simulink subsystem "sdf_node"  (R2022b)
settings: Solver=VariableStepAuto  StartTime=0.0  StopTime=10.0  RelTol=1e-3
model mask{Parameter1=0, Parameter2=0, Parameter3=0, Parameter4=0}
  mask prompts: Parameter1 "alpha"; Parameter2 "beta"; Parameter3 "k"; Parameter4 "Accumulator"
settings Model: Creator=1111293  LastModifiedBy=qaztr
settings SolverCC: AlgebraicLoopSolver=TrustRegion
settings DebuggingCC: UnconnectedInputMsg=warning  UnconnectedOutputMsg=warning  UnconnectedLineMsg=warning  SFMachineParentedDataDiag=warning
settings ModelReferenceCC: EnableRefExpFcnMdlSchedulingChecks=on
settings RTWCC: DLArmComputeVersion=19.05

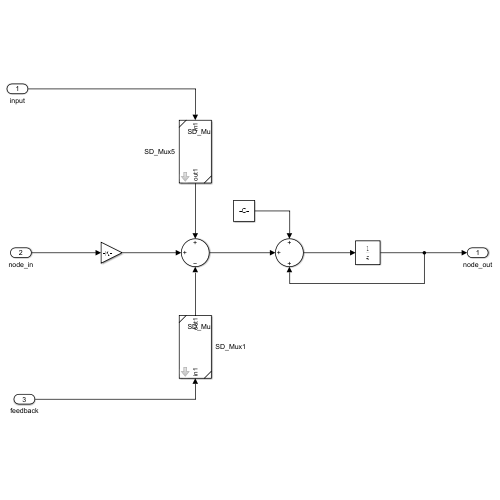
[thumbnail: Simulink's stored preview of the top-level diagram]
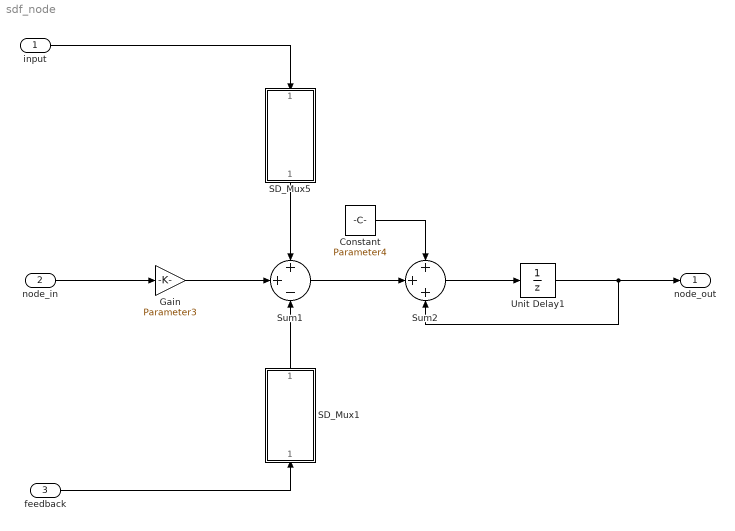
== system sdf_node ==
  input : Inport
  node_in : Inport  Port=2
  feedback : Inport  Port=3
  Constant : Constant  Value=Parameter4
  Gain : Gain  Gain=Parameter3  RndMeth=Round
  SD_Mux1 : Subsystem  ReferencedSubsystem=SD_Mux  a=Parameter1  Parameter2=Inherit: Inherit via internal rule
  SD_Mux5 : Subsystem  ReferencedSubsystem=SD_Mux  a=Parameter2  Parameter2=Inherit: Inherit via internal rule
  Sum1 : Sum  Inputs=++-  OutDataTypeStr=Inherit: Same as accumulator
  Sum2 : Sum  Inputs=+++  OutDataTypeStr=Inherit: Same as accumulator
  Unit Delay1 : UnitDelay  SampleTime=-1  HasFrameUpgradeWarning=on
  node_out : Outport
  wires:
  Unit Delay1/1 -> node_out/1, Sum2/3
  node_in/1 -> Gain/1
  feedback/1 -> SD_Mux1/1
  input/1 -> SD_Mux5/1
  Sum2/1 -> Unit Delay1/1
  SD_Mux1/1 -> Sum1/3
  SD_Mux5/1 -> Sum1/1
  Gain/1 -> Sum1/2
  Sum1/1 -> Sum2/2
  Constant/1 -> Sum2/1
